simulink library "HeliLibrary"  (R2019b)
settings: Solver=ode45  StartTime=0.0  StopTime=10.0  RelTol=1e-3  EnableMultiTasking=on
settings Model: Creator=bpotter  LastModifiedBy=bpotter
settings DataIOCC: LimitDataPoints=on  SaveFormat=Array
settings OptimizationCC: LifeSpan=inf
settings DebuggingCC: AllowSymbolicDim=off  PregeneratedLibrarySubsystemCodeDiagnostic=none  SFUnexpectedBacktrackingDiag=warning  SFNoUnconditionalDefaultTransitionDiag=warning  SFExecutionAtInitializationDiag=none  ArithmeticOperatorsInVariantConditions=warning
settings HardwareCC: ProdBitPerPointer=32  ProdBitPerSizeT=32  ProdBitPerPtrDiffT=32  ProdLargestAtomicFloat=None  ProdIntDivRoundTo=Undefined  ProdEndianess=Unspecified  ProdWordSize=32  ProdHWDeviceType=32-bit Generic
settings ModelReferenceCC: PropagateSignalLabelsOutOfModel=off
settings SFSimCC: SimUseLocalCustomCode=off  CustomCodeUndefinedFunction=UseInterfaceOnly
settings RTWCC: RTWUseLocalCustomCode=off
settings CodeAppCC: StateflowObjectComments=on
settings GRTTargetCC: TargetLangStandard=C89/C90 (ANSI)  GeneratePreprocessorConditionals=Disable all
settings ConfigComp: CovMetricSettings=dw  CovHtmlReporting=on  CovSaveCumulativeToWorkspaceVar=on  CovSaveSingleToWorkspaceVar=on  CovExternalEMLEnable=off

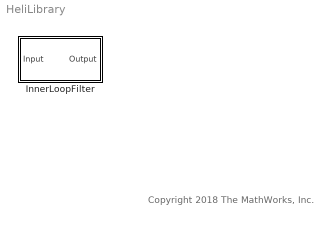
== system HeliLibrary ==
  note: Copyright 2018 The MathWorks, Inc.
  InnerLoopFilter : Subsystem  Tag=FilterWizardSubSystem  RTWFcnName=InnerLoopFilter
      settings: AttributesFormatString=@100Hz  ErrorFcn=dspFilterRealizedInBasicElemsAlgLoopErrFcnCallback  RTWFcnNameOpts=User specified
      mask Display: dpoly([0 40],[1 40]);

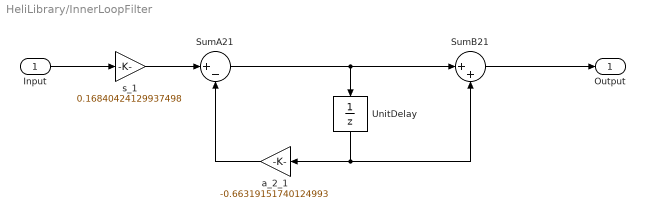
== system HeliLibrary/InnerLoopFilter ==
  Input : Inport
  SumA21 : Sum  Inputs=|+-  RndMeth=Zero  SaturateOnIntegerOverflow=on  OutDataTypeStr=Inherit: Same as first input
  SumB21 : Sum  Inputs=|++  RndMeth=Zero  SaturateOnIntegerOverflow=on  OutDataTypeStr=Inherit: Same as first input
  UnitDelay : UnitDelay  SampleTime=-1  HasFrameUpgradeWarning=on
  a_2_1 : Gain  Gain=-0.66319151740124993  ParamDataTypeStr=double  RndMeth=Zero  SaturateOnIntegerOverflow=on  OutDataTypeStr=Inherit: Same as input
  s_1 : Gain  Gain=0.16840424129937498  ParamDataTypeStr=double  RndMeth=Zero  SaturateOnIntegerOverflow=on  OutDataTypeStr=Inherit: Same as input
  Output : Outport  VectorParamsAs1DForOutWhenUnconnected=off
  wires:
  UnitDelay/1 -> SumB21/2, a_2_1/1
  a_2_1/1 -> SumA21/2
  SumB21/1 -> Output/1
  SumA21/1 -> UnitDelay/1, SumB21/1
  s_1/1 -> SumA21/1
  Input/1 -> s_1/1
